simulink model "tracking_sim_template"  (R2017b)
settings: Solver=VariableStepAuto  StartTime=0.0  StopTime=tF(end, 1)  RelTol=1e-3
values from neighbouring files (symbols this model uses):
  A_x = 1.0    (= 1)    [path_tracking_template.m]
  A_y = 1.0    (= 1)    [path_tracking_template.m]
  F_x_minmax = 0.1    [path_tracking_template.m]
  F_y_minmax = 0.25    [path_tracking_template.m]
  phi_x = pi/2.0    (= 1.57079632679)    [path_tracking_template.m]
  phi_y = pi/4.0    (= 0.785398163397)    [path_tracking_template.m]
libraries: simulink x1
settings Model: Creator=Mrochen  LastModifiedBy=Mrochen

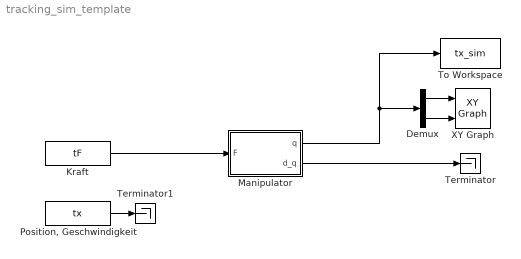
== system tracking_sim_template ==
  Demux : Demux  Outputs=2
  Kraft : FromWorkspace  VariableName=tF  SampleTime=0  OutputAfterFinalValue=Holding final value
  Manipulator : Subsystem
  "Position, Geschwindigkeit" : FromWorkspace  VariableName=tx  SampleTime=0  OutputAfterFinalValue=Holding final value
  Terminator : Terminator
  Terminator1 : Terminator
  To Workspace : ToWorkspace  VariableName=tx_sim  SaveFormat=Timeseries  SampleTime=-1
  XY Graph : simulink/Sinks/XY Graph  xmin=-1.2  xmax=1.2  ymin=-1.2  ymax=1.2  st=-1
  wires:
  Demux/2 -> XY Graph/2
  Demux/1 -> XY Graph/1
  Manipulator/1(q) -> To Workspace/1, Demux/1
  Kraft/1 -> Manipulator/1(F)
  "Position, Geschwindigkeit"/1 -> Terminator1/1
  Manipulator/2(d_q) -> Terminator/1

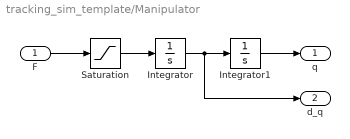
== system tracking_sim_template/Manipulator ==
  F : Inport
  Integrator : Integrator  InitialCondition=[0; 0]
  Integrator1 : Integrator  InitialCondition=[A_x*sin(phi_x); A_y*sin(phi_y)]
  Saturation : Saturate  UpperLimit=[F_x_minmax; F_y_minmax]  LowerLimit=[-F_x_minmax; -F_y_minmax]
  q : Outport
  d_q : Outport  Port=2
  wires:
  F/1 -> Saturation/1
  Integrator1/1 -> q/1
  Integrator/1 -> d_q/1, Integrator1/1
  Saturation/1 -> Integrator/1
